simulink model "simDiagram"  (Simulink 7.6)
settings: Solver=ode45  StartTime=0.0  StopTime=simtime  FixedStep=0.001  RelTol=1e-10  AbsTol=1e-10
values from neighbouring files (symbols this model uses):
  A_Veq = 0.04    [init.m]
  AFR_high = 22    [init.m]
  AFR_low = 8.0    (= 8)    [init.m]
  bsr_max = 0.7    [init.m]
  c_d = 0.9    [init.m]
  c_pa = 1005    [init.m]
  c_pe = 1117    [init.m]
  Chat_T = (1-t_d)*KTTi*rho_w*D^4*(N_mcr/60)^2/Vmax^2    [init.m]
  D = 6.5    [init.m]
  d_c = 0.5    [init.m]
  d_t = 0.5    [init.m]
  eta_em = 1    [init.m]
  eta_ic = 0.98    [init.m]
  eta_t_max = 0.82    [init.m]
  H_l = 40640*10^3    (= 40640000)    [init.m]
  J = 0:0.01:0.74    [init.m]
  J_tc = 1.5*4.83    (= 7.245)    [init.m]
  J_tot = J_tot + J_ew    (= 67447.4931834)    [init.m]
  k_a = 1.4    [init.m]
  k_e = 1.34    [init.m]    (also in tmap.m)
  k_f = [k_f2 k_f1 k_f0]    [init.m]
  k_flw = [1 -0.203493859796 0.693772813684 -0.747867845034 0.372206576043 -11.0504967628 27.5086832027 -10.4699673169 1 1 1 5.5615818662 ... (15 elements, 15x1)]    [cflw.mat]    (also in cmap_flw.m = lsqcurvefit(@compflw,k0,PRvec,Qvec,[],[],options,U2vec))
  K_Q = zeros(size(J))    [init.m]
  k_scv = [0.5, 1, 1.2, 2.0]    [init.m]
  k_srg = [4.5895*10^-5, 0.0018, -0.0645]    [init.m]
  k_t = 2    [init.m]
  K_T = zeros(size(J))    [init.m]
  k_trb = [0.390435968423 -3.37920398425]    [tflw.mat]    (also in tmap.m = lsqcurvefit(@turbflw,k0,PR_t,Q_t))
  k_trq = [0.4, 1, 0.4, 0.8]    [init.m]
  k_z = [k_z1 k_z0]    [init.m]
  Ki = 0.1    [init.m]
  Kp = 1    [init.m]
  Kw = 1    [init.m]
  M_a = 0.25*M_s    (= 1589500)    [init.m]
  m_fmax = 0.0393    [init.m]
  M_s = 6.358*10^6    (= 6358000)    [init.m]
  N_mcr = 114.6    [init.m]
  p = [0.328077427849 -0.26658012165 1.54534042269 -0.0646814508145 0.804569801172 -2.25026225382 0.013357862542 -0.101778856641 0.0321254948084 0.563804002916 -0.0020574891572 0.0210610050218 ... (21 elements, 1x21)]    [ceff.mat]    (also in ceff_ABB_TPL_B.mat = [3.8647104441 -0.945126326208 1.79579254622 0.0101929790733 ; cmap_eff.m = coeffvalues(eta); cmap_flw.m = polyfit(M, Psi_plot, 5))
  p_amb = 101325    [init.m]
  p_imax = 16*10^5    (= 1600000)    [init.m]
  Pi_tr = 0.95    [init.m]
  R_a = 287    [init.m]
  R_e = 277.1    [init.m]
  rho_a = 1.23    [init.m]
  rho_w = 1025    [init.m]
  T_amb = 293.2    [init.m]
  t_d = 0.2    [init.m]
  T_ep = 273+230    (= 503)    [init.m]    (also in simRun.m = interm(:,15))
  T_water = 298    [init.m]
  u_0 = 1    [init.m]
  u_lb = 0    [init.m]
  u_ub = 1    [init.m]
  V_d = 0.5429    [init.m]
  V_em = 1.5*V_d    (= 0.81435)    [init.m]
  V_im = 1.5*V_d    (= 0.81435)    [init.m]
  V_s0 = 15*0.5144    (= 7.716)    [init.m]
  w = 0.277    [init.m]    (also in simRun.m = simout.get('w'))
  x0 = [p_im0; T_im0; p_em0; T_em0; w_tc0; w_e0]    [init.m]
  z_c = 6    [init.m]
undefined symbols (not defined in the file or in its folder): sigbuilder_block
libraries: simulink x2
settings Model: Creator=andrkar  LastModifiedBy=andrkar

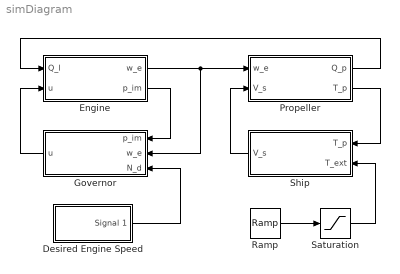
== system simDiagram ==
  Desired Engine Speed : Subsystem  Tag=STV Subsys  LoadFcn=sigbuilder_block('load');  StartFcn=sigbuilder_block('start');  StopFcn=sigbuilder_block('stop');  ClipboardFcn=sigbuilder_block('clipboard');  mask(Sigbuilder block){}
      mask help: Create and generate interchangeable groups of signals whose waveforms are piecewise linear.
      mask init:
      | if ~strcmp(get_param(bdroot(gcbh),'SimulationStatus'),'stopped') tuvar = sigbuilder_block('maskInit'); end
      settings: CopyFcn=sigbuilder_block('copy');  DeleteFcn=sigbuilder_block('delete');  ModelCloseFcn=sigbuilder_block('modelClose');  PreSaveFcn=sigbuilder_block('preSave');  NameChangeFcn=sigbuilder_block('namechange');  OpenFcn=sigbuilder_block('open',[168 213 550.5 399.75 ]);  CloseFcn=sigbuilder_block('close');
      mask Display: plot(0,0,100,100,[10,10,40,40,10],[80,20,20,80,80],[40,10],[50,50], [40,27,10],[65,72,56],[40,25,25,10],[28,28,43,43]);
  Engine : Subsystem
  Governor : Subsystem
  Propeller : Subsystem
  Ramp : simulink/Sources/Ramp  SystemSampleTime=-1  slope=1666.67  start=120  X0=0
  Saturation : Saturate  UpperLimit=100000  LowerLimit=0
  Ship : Subsystem
  wires:
  Engine/1(w_e) -> Propeller/1(w_e), Governor/2(w_e)
  Ship/1(V_s) -> Propeller/2(V_s)
  Propeller/2(T_p) -> Ship/1(T_p)
  Ramp/1 -> Saturation/1
  Engine/2(p_im) -> Governor/1(p_im)
  Governor/1(u) -> Engine/2(u)
  Desired Engine Speed/1(Signal 1) -> Governor/3(N_d)
  Saturation/1 -> Ship/2(T_ext)
  Propeller/1(Q_p) -> Engine/1(Q_l)

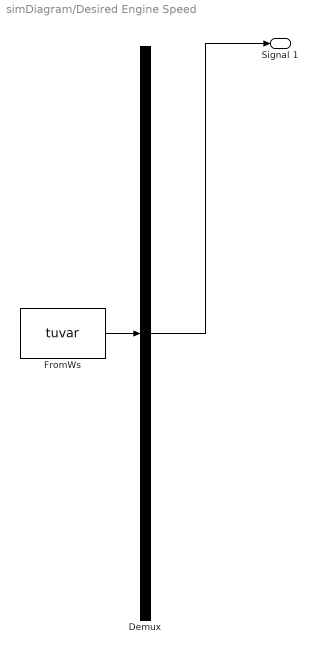
== system simDiagram/Desired Engine Speed ==
  Demux : Demux  Tag=STV Demux  Outputs=1
  FromWs : FromWorkspace  Tag=STV FromWs  VariableName=tuvar  SampleTime=0  SigBuilderData=DataTag0  VnvData=DataTag1
      SigBuilderData=|
      | common.afterFinalStr = 'Extrapolate'
      | common.sampleTime = 0
      | dataSet.timeRange = [0 1000]
      | dataSet.name = 'Group 1'
      | sbobj.Groups.Name = 'Group 1'
      | sbobj.Groups.Signals.Name = 'Signal 1'
      | sbobj.Groups.Signals.XData = [0 360 480 740 800 1000]
      | sbobj.Groups.Signals.YData = [114.4 114.4 85 85 104.8 104.9]
      | sbobj.Groups.TimeRange = [0 1000]
  Signal 1 : Outport  Tag=STV Outport
  wires:
  Demux/1 -> Signal 1/1
  FromWs/1 -> Demux/1

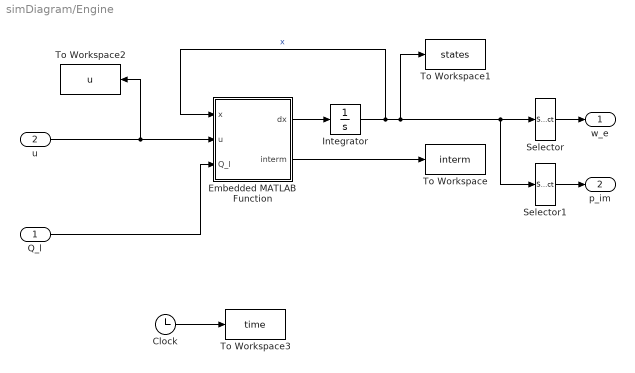
== system simDiagram/Engine ==
  Q_l : Inport
  u : Inport  Port=2
  Clock : Clock
      settings: Decimation=10
  Embedded MATLAB Function : Stateflow chart  TreatAsAtomicUnit=on
  Integrator : Integrator  InitialCondition=x0
  Selector : Selector  InputPortWidth=6  IndexOptions=Index vector (dialog)  Indices=[6]  OutputSizes=1
  Selector1 : Selector  InputPortWidth=6  IndexOptions=Index vector (dialog)  Indices=[1]  OutputSizes=1
  To Workspace : ToWorkspace  VariableName=interm  SampleTime=-1  SaveFormat=Array
  To Workspace1 : ToWorkspace  VariableName=states  SampleTime=-1  SaveFormat=Array
  To Workspace2 : ToWorkspace  VariableName=u  SampleTime=-1  SaveFormat=Array
  To Workspace3 : ToWorkspace  VariableName=time  SampleTime=-1  SaveFormat=Array
  w_e : Outport
  p_im : Outport  Port=2
  wires:
  Integrator/1 -> Embedded MATLAB Function/1(x), To Workspace1/1, Selector/1, Selector1/1  "x"
  Embedded MATLAB Function/1(dx) -> Integrator/1
  Embedded MATLAB Function/2(interm) -> To Workspace/1
  Q_l/1 -> Embedded MATLAB Function/3(Q_l)
  Selector/1 -> w_e/1
  Selector1/1 -> p_im/1
  Clock/1 -> To Workspace3/1
  u/1 -> Embedded MATLAB Function/2(u), To Workspace2/1

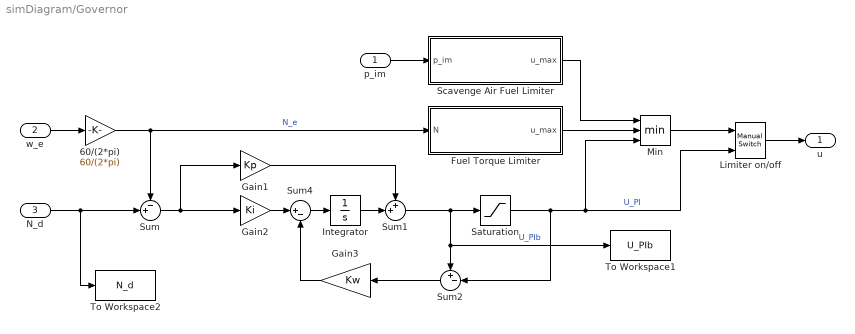
== system simDiagram/Governor ==
  p_im : Inport
  w_e : Inport  Port=2
  N_d : Inport  Port=3
  60/(2*pi) : Gain  Gain=60/(2*pi)
  Fuel Torque Limiter : Stateflow chart  TreatAsAtomicUnit=on
  Gain1 : Gain  Gain=Kp
  Gain2 : Gain  Gain=Ki
  Gain3 : Gain  Gain=Kw
  Integrator : Integrator  InitialCondition=u_0
  Limiter on/off : simulink/Signal Routing/Manual Switch  SystemSampleTime=-1  sw=1  action=0  varsize=off
  Min : MinMax  Inputs=3
  Saturation : Saturate  UpperLimit=u_ub  LowerLimit=u_lb
  Scavenge Air Fuel Limiter : Stateflow chart  TreatAsAtomicUnit=on
  Sum : Sum  Inputs=-+|
  Sum1 : Sum  Inputs=++|
  Sum2 : Sum  Inputs=+-|
  Sum4 : Sum  Inputs=|+-
  To Workspace1 : ToWorkspace  VariableName=U_PIb  SampleTime=-1  SaveFormat=Array
  To Workspace2 : ToWorkspace  VariableName=N_d  SampleTime=-1  SaveFormat=Array
  u : Outport
  wires:
  w_e/1 -> 60/(2*pi)/1
  Sum/1 -> Gain1/1, Gain2/1
  Gain1/1 -> Sum1/1
  Integrator/1 -> Sum1/2
  Sum1/1 -> Saturation/1, Sum2/1, To Workspace1/1  "U_PIb"
  Saturation/1 -> Sum2/2, Limiter on/off/2, Min/3  "U_PI"
  Gain2/1 -> Sum4/1
  Sum4/1 -> Integrator/1
  Sum2/1 -> Gain3/1
  Gain3/1 -> Sum4/2
  60/(2*pi)/1 -> Sum/1, Fuel Torque Limiter/1(N)  "N_e"
  N_d/1 -> Sum/2, To Workspace2/1
  p_im/1 -> Scavenge Air Fuel Limiter/1(p_im)
  Min/1 -> Limiter on/off/1
  Limiter on/off/1 -> u/1
  Scavenge Air Fuel Limiter/1(u_max) -> Min/1
  Fuel Torque Limiter/1(u_max) -> Min/2

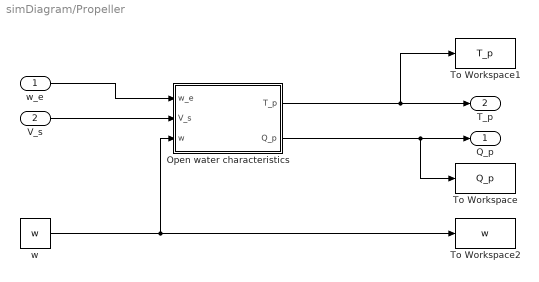
== system simDiagram/Propeller ==
  w_e : Inport
  V_s : Inport  Port=2
  Open water characteristics : Stateflow chart  TreatAsAtomicUnit=on
  To Workspace : ToWorkspace  VariableName=Q_p  SampleTime=-1  SaveFormat=Array
  To Workspace1 : ToWorkspace  VariableName=T_p  SampleTime=-1  SaveFormat=Array
  To Workspace2 : ToWorkspace  VariableName=w  SampleTime=-1  SaveFormat=Array
  w : Constant  Value=w
  Q_p : Outport
  T_p : Outport  Port=2
  wires:
  w_e/1 -> Open water characteristics/1(w_e)
  V_s/1 -> Open water characteristics/2(V_s)
  w/1 -> Open water characteristics/3(w), To Workspace2/1
  Open water characteristics/1(T_p) -> T_p/1, To Workspace1/1
  Open water characteristics/2(Q_p) -> Q_p/1, To Workspace/1

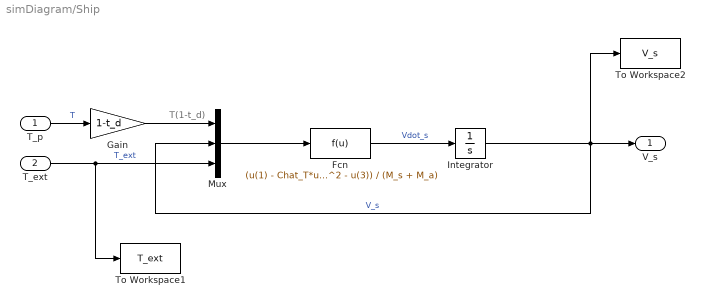
== system simDiagram/Ship ==
  note: T(1-t_d)
  T_p : Inport
  T_ext : Inport  Port=2
  Fcn : Fcn  Expr=(u(1) - Chat_T*u(2)^2 - u(3)) / (M_s + M_a)
  Gain : Gain  Gain=1-t_d
  Integrator : Integrator  InitialCondition=V_s0
  Mux : Mux  Inputs=3
  To Workspace1 : ToWorkspace  VariableName=T_ext  SampleTime=-1  SaveFormat=Array
  To Workspace2 : ToWorkspace  VariableName=V_s  SampleTime=-1  SaveFormat=Array
  V_s : Outport
  wires:
  Fcn/1 -> Integrator/1  "Vdot_s"
  Integrator/1 -> Mux/2, V_s/1, To Workspace2/1  "V_s"
  T_p/1 -> Gain/1  "T"
  Mux/1 -> Fcn/1
  Gain/1 -> Mux/1
  T_ext/1 -> Mux/3, To Workspace1/1  "T_ext"

== matlab function Engine/Embedded MATLAB Function ==
  data: dx output double; x input double; u input double; Q_l input double; m_fmax parameter double; c_d parameter double; A_Veq parameter double; k_t parameter double; d_t parameter double; eta_t_max parameter double; bsr_max parameter double; eta_em parameter double; J_tot parameter double; V_im parameter double; V_em parameter double; k_a parameter double; k_e parameter double; R_a parameter double; R_e parameter double; J_tc parameter double; z_c parameter double; V_d parameter double; k_f parameter double; p_imax parameter double; T_amb parameter double; p_amb parameter double; c_pa parameter double; c_pe parameter double; AFR_low parameter double; AFR_high parameter double; H_l parameter double; k_z parameter double; rho_a parameter double; interm output double; p parameter double; d_c parameter double; k_flw parameter double; k_trb parameter double; Pi_tr parameter double; T_water parameter double; eta_ic parameter double; k_srg parameter double; T_ep parameter double
function [dx,interm]= engine(x,u,Q_l,m_fmax,c_d,A_Veq,k_t,d_t,eta_t_max,bsr_max,eta_em,J_tot,V_im,V_em,k_a,k_e,R_a,R_e,J_tc,z_c,V_d,k_f,p_imax,T_amb,p_amb,c_pa, c_pe,AFR_low,AFR_high,H_l,k_z,rho_a,p,d_c,k_flw,k_trb, Pi_tr, T_water, eta_ic, k_srg, T_ep)

% [dx,interm] = ENGINE(x,u,Q_l,...); 
%   Calulates the differential equations to simulate the engine.
%
%   Data:
%       x   : column vector of engine states, x = [p_im; T_im; p_em; T_em; w_tc; w_e]
%       u   : fuel rack position
%       Q_l : propeller load torque
%       ... : parameters used in the script
%   Output:
%       dx  : the calculated differential equations of x
%       interm: intermediate / plotting variables
%%

% Defining the size of the output vectors
dx = zeros(length(x),1);
interm = zeros(25,1);

p_im = x(1);
T_im = x(2);
p_em = x(3);
T_em = x(4);
w_tc = x(5);
w_e = x(6);

% Compressor
Uc = 0.5*d_c*w_tc;  % Compressor impeller tip speed [m/s]
if p_im < p_amb     % To avoid negative pressure in intake manifold, should be removed?
    p_im = p_amb;
end
Q = compflwEmbedded(k_flw,p_im/p_amb,Uc,k_a,R_a,T_amb,c_pa,d_c);    % Compressor volume flow rate [m^3/s]
Q_srg = k_srg(1)*Uc^2 + k_srg(2)*Uc + k_srg(3);                     % Surge line volume flow rate [m^3/s]
Q = max(Q,Q_srg);                                                   % Surge is neglected                                                              
mdot_c = Q * rho_a;                                                 % Compressor mass flow rate [kg/s]

x = Q;
y = p_im/p_amb;
eta_c = p(1) + p(2)*x + p(3)*y + p(4)*x^2 + p(5)*x*y + p(6)*y^2 + p(7)*x^3 + p(8)*x^2*y + p(9)*x*y^2 + p(10)*y^3 + p(11)*x^4 + p(12)*x^3*y + p(13)*x^2*y^2 + p(14)*x*y^3 + p(15)*y^4 + p(16)*x^5 + p(17)*x^4*y + p(18)*x^3*y^2 + p(19)*x^2*y^3 + p(20)*x*y^4 + p(21)*y^5; % Compressor efficiency
eta_c = max(eta_c,0); % Efficiency can not be negative

T_c = T_amb + (T_amb / eta_c)*((p_im/p_amb)^((k_a-1)/k_a)-1);       % Temperature after compressor [K]
T_i = (1 - eta_ic)*T_c + eta_ic * T_water;                          % Temperature after intercooler [K]

% %Massflow of air through engine (Lipschitz)
% Pi = p_em / p_im;
% Psi_tr = Pi_tr^(1/k_a) * sqrt((2*k_a/(k_a-1))*(1-Pi_tr^((k_a-1)/k_a))); % calc i init i stedet?
% dPi = 0.0000001;
% dy = (Pi_tr+dPi)^(1/k_a)*sqrt((2*k_a/(k_a-1))*(1-(Pi_tr+dPi)^((k_a-1)/k_a))) - Pi_tr^(1/k_a)*sqrt((2*k_a/(k_a-1))*(1-Pi_tr^((k_a-1)/k_a)));
% a = ((dy/dPi)*(Pi_tr-1) - Psi_tr) / (2*(Pi_tr-1)^3);
% b = dy/dPi - 3*a*(Pi_tr-1)^2;
% 
% p_cr = (2/(k_a+1))^(k_a/(k_a-1))*p_im;
% if p_em < p_cr
%     Psi_e = sqrt(k_a*(2/(k_a+1))^((k_a+1)/(k_a-1)));
% else
%     if Pi < Pi_tr % To avoid complex numbers.
%         Psi_e = (p_em/p_im)^(1/k_a)*sqrt((2*k_a/(k_a-1))*(1-(p_em/p_im)^((k_a-1)/k_a)));
%     else
%         Psi_e = a*(Pi-1)^3 + b*(Pi-1);
%     end
% end
% mdot_a = (c_d * A_Veq * p_im)/sqrt(R_a*T_im)*Psi_e;

% Massflow of air through engine
p_cr = (2/(k_a+1))^(k_a/(k_a-1))*p_im;
if p_em < p_cr
    Psi_e = sqrt(k_a*(2/(k_a+1))^((k_a+1)/(k_a-1)));
else
    if p_em > p_im  % To avoid complex numbers, remove? 
        Psi_e = 0;
    else
        Psi_e = (p_em/p_im)^(1/k_a)*sqrt((2*k_a/(k_a-1))*(1-(p_em/p_im)^((k_a-1)/k_a)));
    end
end
mdot_a = (c_d * A_Veq * p_im)/sqrt(R_a*T_im)*Psi_e; % Air mass flow rate through engine cylinders [kg/s]

% Engine cylinders
m_f = z_c * m_fmax * u;         % Fuel injected in cylinders per cycle [kg]
mdot_f = (m_f*w_e) / (2*pi);    % Mass flow rate of fuel injected in cylinders [kg/s]
mdot_e = mdot_a + mdot_f;       % Exhaust gas mass flow rate from cylinders to exhaust manifold[kg/s]
AFR = mdot_a / mdot_f;          % Air-to-fuel ratio
if AFR >= AFR_high              % Calculating combustion/thermodynamical efficiency in the cylinders
    eta_th = 1;
elseif AFR <= AFR_low
    eta_th = 0;
else
    eta_th = (AFR-AFR_low)/(AFR_high - AFR_low);
end
p_i = eta_th*p_imax*u;                  % Indicated mean effective pressure [Pa]
N_e = (60/(2*pi))*w_e;                  % Engine speed [rpm]
p_f = k_f(1)*p_i + k_f(2)*N_e + k_f(3); % Friction mean effective pressure [Pa]
p_e = p_i - p_f;                        % Break mean effective pressure [Pa]
p_e = max(p_e,0);                       % Can not have negative bmep. Happens if AFR<AFR_min giving p_i = 0 and p_f > 0.
zeta = k_z(1)*p_e + k_z(2);             % Fuel hemical energy proportien left in exhaust gas
T_e = (mdot_a*c_pa*T_im+mdot_f*H_l*zeta)/(mdot_e*c_pe) * eta_em; % Temperature of exhaust gas into exhaust manifold [K]
Q_e = (p_e * z_c * V_d) / (2*pi);       % Engine torque [Nm]

% Exhaust Pipe
p_ep = p_amb;   % Exhaust pipe pressure [Pa]
%T_ep = 273+230; % Exhaust pipe temperature [K]

% Turbine
mdot_t = k_trb(1)*sqrt(1-(p_em/p_ep)^k_trb(2)) * sqrt(T_em) * p_em/(R_e*T_em);  % Turbine massflow [kg/s]
bsr = (0.5*d_t*w_tc) / (sqrt(2*c_pe*T_em*(1-(p_ep/p_em)^((k_e-1)/k_e))));       % Turbine blade speed ratio
eta_t = eta_t_max*(1 - k_t*(bsr-bsr_max)^2);                                    % Turbine efficiency
eta_t = max(eta_t,0);                                                           % Negative efficiency not allowed

% Turbocharger   
P_c = (1/eta_c)*mdot_c*c_pa*(T_c-T_amb);    % Compressor absorbed power [W]
P_t = eta_t*mdot_t*c_pe*(T_em-T_ep);        % Turbine produced power [W]
Q_c = P_c / w_tc;                           % Compressor absorbed torque [Nm]
Q_t = P_t / w_tc;                           % Turbine produced torque [Nm]    

%% Calculation of dynamic variables
%Intake manifold
dp_im = ((k_a*R_a)/V_im)*(mdot_c*T_i - mdot_a*T_im);
dT_im = ((R_a*T_im)/(p_im*V_im))*(k_a*T_i*mdot_c - k_a*T_im*mdot_a - T_im*(mdot_c-mdot_a));

%Exhaust manifold
dp_em = ((k_e*R_e)/V_em)*(mdot_e*T_e - mdot_t*T_em);
dT_em = ((R_e*T_em)/(p_em*V_em))*(k_e*T_e*mdot_e - k_e*T_em*mdot_t - T_em*(mdot_e-mdot_t));

%Turbocharger Dynamics
dw_tc = (Q_t - Q_c) / J_tc;

%Crankshaft Dynamics
dw_e = (Q_e - Q_l) / J_tot;

%% Output
dx = [dp_im; dT_im; dp_em; dT_em; dw_tc; dw_e];
interm = [T_c mdot_c mdot_a m_f mdot_f mdot_e AFR eta_th p_i p_f p_e zeta T_e p_ep T_ep mdot_t Q_c Q_t Q_e Q_l bsr eta_t eta_c Psi_e T_i]';

end

== matlab function Propeller/Open water characteristics ==
  data: T_p output double; w_e input double; V_s input double; w input double; Q_p output double; K_Q parameter double; K_T parameter double; J parameter double; D parameter double; rho_w parameter double
function [T_p,Q_p] = prop(w_e,V_s,w,K_Q,K_T,J,D,rho_w) %#eml

n = w_e / (2*pi);   % Propeller speed [rps]

V_a = (1-w)*V_s;    % Advance speed [m/s]
J_a = V_a / (n*D);

% Calculates the torque and thrust coefficients for the given advance speed
K_Ti = interp1(J,K_T,J_a,'linear');
K_Qi = interp1(J,K_Q,J_a,'linear'); 

% Calculates the nominal thrust and torque
T_p = K_Ti * rho_w * n^2 * D^4;
Q_p = K_Qi * rho_w * n^2 * D^5;

== matlab function Governor/Fuel Torque Limiter ==
  data: N input double; u_max output double; N_mcr parameter double; k_trq parameter double
function u_max = torqueLim(N,N_mcr,k_trq)
% TORQUELIM 
%   
%   Detailed explanation goes here

a = k_trq(1);
b = k_trq(2);
c = k_trq(3);
d = k_trq(4);

e = (b-a) / (d-c);
f = b - d*e;

if N <= c*N_mcr
    u_max = a;
elseif N >= d*N_mcr
    u_max = b;
else
    u_max = e*(N/N_mcr) + f;
end

end

== matlab function Governor/Scavenge Air Fuel Limiter ==
  data: p_im input double; u_max output double; k_scv parameter double; p_amb parameter double
function u_max = scavLim(p_im,k_scv,p_amb)
% SCAVLIM(N,N_mcr,k_scv) 
%   
%   Detailed explanation goes here

a = k_scv(1);
b = k_scv(2);
c = k_scv(3);
d = k_scv(4);

e = (b-a) / (d-c);
f = b - d*e;

if p_im/p_amb <= c
    u_max = a;
elseif p_im/p_amb >= d
    u_max = b;
else
    u_max = e*(p_im/p_amb) + f;
end

end
